simulink model "case8"  (R2024b)
settings: Solver=FixedStepAuto  StartTime=0  StopTime=1  FixedStep=1e-7  RelTol=1e-3
values from neighbouring files (symbols this model uses):
  SG_D_1_D = 0.01056    [IEEE9_case_parameters.m]    (also in case1_parameters.m; case2_parameters.m; case3_parameters.m; case4_parameters.m)
  SG_D_1_EnableSaturation = 0    [IEEE9_case_parameters.m]    (also in case1_parameters.m; case2_parameters.m; case3_parameters.m; case4_parameters.m)
  SG_D_1_f0 = 60    [IEEE9_case_parameters.m]    (also in case1_parameters.m; case2_parameters.m; case3_parameters.m; case4_parameters.m)
  SG_D_1_H = 7.5    [IEEE9_case_parameters.m]    (also in case1_parameters.m; case2_parameters.m; case3_parameters.m; case4_parameters.m)
  SG_D_1_K_A = 20    [IEEE9_case_parameters.m]    (also in case1_parameters.m; case2_parameters.m; case3_parameters.m; case4_parameters.m)
  SG_D_1_K_E = 1.000000e+1    (= 10)    [IEEE9_case_parameters.m]    (also in case1_parameters.m; case2_parameters.m; case3_parameters.m; case4_parameters.m)
  SG_D_1_K_F = 2.363    [IEEE9_case_parameters.m]    (also in case1_parameters.m; case2_parameters.m; case3_parameters.m; case4_parameters.m)
  SG_D_1_K_s = 0.5    [IEEE9_case_parameters.m]    (also in case1_parameters.m = 5; case2_parameters.m = 5; case3_parameters.m = 5; case4_parameters.m = 5)
  SG_D_1_R_a = 0.001088    [IEEE9_case_parameters.m]    (also in case1_parameters.m; case2_parameters.m; case3_parameters.m; case4_parameters.m)
  SG_D_1_S_A = 1    [IEEE9_case_parameters.m]    (also in case1_parameters.m; case2_parameters.m; case3_parameters.m; case4_parameters.m)
  SG_D_1_S_B = 0.103    [IEEE9_case_parameters.m]    (also in case1_parameters.m; case2_parameters.m; case3_parameters.m; case4_parameters.m)
  SG_D_1_S_N = 10.659857    [IEEE9_case_parameters.m]    (also in case1_parameters.m; case2_parameters.m; case3_parameters.m; case4_parameters.m)
  SG_D_1_SpeedPara = 200    [IEEE9_case_parameters.m]    (also in case1_parameters.m; case2_parameters.m; case3_parameters.m; case4_parameters.m)
  SG_D_1_T_0 = 0.720173    [IEEE9_case_parameters.m]    (also in case1_parameters.m = 0.755522; case2_parameters.m = 0.808931; case3_parameters.m = 0.869402; case4_parameters.m = 0.729316)
  SG_D_1_T_1 = 0.3    [IEEE9_case_parameters.m]    (also in case1_parameters.m; case2_parameters.m; case3_parameters.m; case4_parameters.m)
  SG_D_1_T_2 = 0.05    [IEEE9_case_parameters.m]    (also in case1_parameters.m; case2_parameters.m; case3_parameters.m; case4_parameters.m)
  SG_D_1_T_3 = 0.02    [IEEE9_case_parameters.m]    (also in case1_parameters.m; case2_parameters.m; case3_parameters.m; case4_parameters.m)
  SG_D_1_T_4 = 0.005    [IEEE9_case_parameters.m]    (also in case1_parameters.m; case2_parameters.m; case3_parameters.m; case4_parameters.m)
  SG_D_1_T_A = 0.02    [IEEE9_case_parameters.m]    (also in case1_parameters.m; case2_parameters.m; case3_parameters.m; case4_parameters.m)
  SG_D_1_T_dd = 8.000000e+0    (= 8)    [IEEE9_case_parameters.m]    (also in case1_parameters.m; case2_parameters.m; case3_parameters.m; case4_parameters.m)
  SG_D_1_T_ddd = 0.04    [IEEE9_case_parameters.m]    (also in case1_parameters.m; case2_parameters.m; case3_parameters.m; case4_parameters.m)
  SG_D_1_T_E = 0.314    [IEEE9_case_parameters.m]    (also in case1_parameters.m; case2_parameters.m; case3_parameters.m; case4_parameters.m)
  SG_D_1_T_F = 0.35    [IEEE9_case_parameters.m]    (also in case1_parameters.m; case2_parameters.m; case3_parameters.m; case4_parameters.m)
  SG_D_1_T_qd = 0.8    [IEEE9_case_parameters.m]    (also in case1_parameters.m; case2_parameters.m; case3_parameters.m; case4_parameters.m)
  SG_D_1_T_qdd = 0.02    [IEEE9_case_parameters.m]    (also in case1_parameters.m; case2_parameters.m; case3_parameters.m; case4_parameters.m)
  SG_D_1_T_speed = 0.1    [IEEE9_case_parameters.m]    (also in case1_parameters.m = 200; case2_parameters.m = 200; case3_parameters.m = 200; case4_parameters.m = 200)
  SG_D_1_T_w = 0.5    [IEEE9_case_parameters.m]    (also in case1_parameters.m; case2_parameters.m; case3_parameters.m; case4_parameters.m)
  SG_D_1_V_ref = 1.990276    [IEEE9_case_parameters.m]    (also in case1_parameters.m = 2.042296; case2_parameters.m = 2.051388; case3_parameters.m = 2.089584; case4_parameters.m = 2.01845)
  SG_D_1_w_ref = 376.991118    [IEEE9_case_parameters.m]    (also in case1_parameters.m; case2_parameters.m; case3_parameters.m; case4_parameters.m)
  SG_D_1_wb = 6.000000e+1    (= 60)    [IEEE9_case_parameters.m]    (also in case1_parameters.m; case2_parameters.m; case3_parameters.m; case4_parameters.m)
  SG_D_1_x_d = 1.9    [IEEE9_case_parameters.m]    (also in case1_parameters.m; case2_parameters.m; case3_parameters.m; case4_parameters.m)
  SG_D_1_x_dd = 0.302    [IEEE9_case_parameters.m]    (also in case1_parameters.m; case2_parameters.m; case3_parameters.m; case4_parameters.m)
  SG_D_1_x_ddd = 0.204    [IEEE9_case_parameters.m]    (also in case1_parameters.m; case2_parameters.m; case3_parameters.m; case4_parameters.m)
  SG_D_1_x_l = 0.05    [IEEE9_case_parameters.m]    (also in case1_parameters.m; case2_parameters.m; case3_parameters.m; case4_parameters.m)
  SG_D_1_x_q = 1.3    [IEEE9_case_parameters.m]    (also in case1_parameters.m; case2_parameters.m; case3_parameters.m; case4_parameters.m)
  SG_D_1_x_qd = 0.5    [IEEE9_case_parameters.m]    (also in case1_parameters.m; case2_parameters.m; case3_parameters.m; case4_parameters.m)
  SG_D_1_x_qdd = 0.3    [IEEE9_case_parameters.m]    (also in case1_parameters.m; case2_parameters.m; case3_parameters.m; case4_parameters.m)
  SG_D_2_D = 0.02    [IEEE9_case_parameters.m]    (also in case1_parameters.m; case2_parameters.m; case3_parameters.m; case4_parameters.m)
  SG_D_2_EnableSaturation = 0    [IEEE9_case_parameters.m]    (also in case1_parameters.m; case2_parameters.m; case3_parameters.m; case4_parameters.m)
  SG_D_2_f0 = 60    [IEEE9_case_parameters.m]    (also in case1_parameters.m; case2_parameters.m; case3_parameters.m; case4_parameters.m)
  SG_D_2_H = 8.000000e+0    (= 8)    [IEEE9_case_parameters.m]    (also in case1_parameters.m; case2_parameters.m; case3_parameters.m; case4_parameters.m)
  SG_D_2_K_A = 20    [IEEE9_case_parameters.m]    (also in case1_parameters.m; case2_parameters.m; case3_parameters.m; case4_parameters.m)
  SG_D_2_K_E = 1.000000e+1    (= 10)    [IEEE9_case_parameters.m]    (also in case1_parameters.m; case2_parameters.m; case3_parameters.m; case4_parameters.m)
  SG_D_2_K_F = 2.363    [IEEE9_case_parameters.m]    (also in case1_parameters.m; case2_parameters.m; case3_parameters.m; case4_parameters.m)
  SG_D_2_K_s = 0.5    [IEEE9_case_parameters.m]    (also in case1_parameters.m = 4; case2_parameters.m = 4; case3_parameters.m = 4; case4_parameters.m = 4)
  SG_D_2_R_a = 0.001088    [IEEE9_case_parameters.m]    (also in case1_parameters.m; case2_parameters.m; case3_parameters.m; case4_parameters.m)
  SG_D_2_S_A = 1    [IEEE9_case_parameters.m]    (also in case1_parameters.m; case2_parameters.m; case3_parameters.m; case4_parameters.m)
  SG_D_2_S_B = 0.103    [IEEE9_case_parameters.m]    (also in case1_parameters.m; case2_parameters.m; case3_parameters.m; case4_parameters.m)
  SG_D_2_S_N = 10.659857    [IEEE9_case_parameters.m]    (also in case1_parameters.m; case2_parameters.m; case3_parameters.m; case4_parameters.m)
  SG_D_2_SpeedPara = 200    [IEEE9_case_parameters.m]    (also in case1_parameters.m; case2_parameters.m; case3_parameters.m; case4_parameters.m)
  SG_D_2_T_0 = 1.632913    [IEEE9_case_parameters.m]    (also in case1_parameters.m = 1.632925; case2_parameters.m = 1.632915; case3_parameters.m = 1.632914; case4_parameters.m = 1.632927)
  SG_D_2_T_1 = 0.2    [IEEE9_case_parameters.m]    (also in case1_parameters.m; case2_parameters.m; case3_parameters.m; case4_parameters.m)
  SG_D_2_T_2 = 0.05    [IEEE9_case_parameters.m]    (also in case1_parameters.m; case2_parameters.m; case3_parameters.m; case4_parameters.m)
  SG_D_2_T_3 = 0.02    [IEEE9_case_parameters.m]    (also in case1_parameters.m; case2_parameters.m; case3_parameters.m; case4_parameters.m)
  SG_D_2_T_4 = 0.005    [IEEE9_case_parameters.m]    (also in case1_parameters.m; case2_parameters.m; case3_parameters.m; case4_parameters.m)
  SG_D_2_T_A = 0.02    [IEEE9_case_parameters.m]    (also in case1_parameters.m; case2_parameters.m; case3_parameters.m; case4_parameters.m)
  SG_D_2_T_dd = 7.9    [IEEE9_case_parameters.m]    (also in case1_parameters.m; case2_parameters.m; case3_parameters.m; case4_parameters.m)
  SG_D_2_T_ddd = 0.04    [IEEE9_case_parameters.m]    (also in case1_parameters.m; case2_parameters.m; case3_parameters.m; case4_parameters.m)
  SG_D_2_T_E = 0.314    [IEEE9_case_parameters.m]    (also in case1_parameters.m; case2_parameters.m; case3_parameters.m; case4_parameters.m)
  SG_D_2_T_F = 0.35    [IEEE9_case_parameters.m]    (also in case1_parameters.m; case2_parameters.m; case3_parameters.m; case4_parameters.m)
  SG_D_2_T_qd = 0.8    [IEEE9_case_parameters.m]    (also in case1_parameters.m; case2_parameters.m; case3_parameters.m; case4_parameters.m)
  SG_D_2_T_qdd = 0.015    [IEEE9_case_parameters.m]    (also in case1_parameters.m; case2_parameters.m; case3_parameters.m; case4_parameters.m)
  SG_D_2_T_speed = 0.1    [IEEE9_case_parameters.m]    (also in case1_parameters.m = 150; case2_parameters.m = 150; case3_parameters.m = 150; case4_parameters.m = 150)
  SG_D_2_T_w = 0.35    [IEEE9_case_parameters.m]    (also in case1_parameters.m; case2_parameters.m; case3_parameters.m; case4_parameters.m)
  SG_D_2_V_ref = 2.58547    [IEEE9_case_parameters.m]    (also in case1_parameters.m = 2.597896; case2_parameters.m = 2.587136; case3_parameters.m = 2.586042; case4_parameters.m = 2.599679)
  SG_D_2_w_ref = 376.991118    [IEEE9_case_parameters.m]    (also in case1_parameters.m; case2_parameters.m; case3_parameters.m; case4_parameters.m)
  SG_D_2_wb = 6.000000e+1    (= 60)    [IEEE9_case_parameters.m]    (also in case1_parameters.m; case2_parameters.m; case3_parameters.m; case4_parameters.m)
  SG_D_2_x_d = 1.8    [IEEE9_case_parameters.m]    (also in case1_parameters.m; case2_parameters.m; case3_parameters.m; case4_parameters.m)
  SG_D_2_x_dd = 0.302    [IEEE9_case_parameters.m]    (also in case1_parameters.m; case2_parameters.m; case3_parameters.m; case4_parameters.m)
  SG_D_2_x_ddd = 0.204    [IEEE9_case_parameters.m]    (also in case1_parameters.m; case2_parameters.m; case3_parameters.m; case4_parameters.m)
  SG_D_2_x_l = 0.05    [IEEE9_case_parameters.m]    (also in case1_parameters.m; case2_parameters.m; case3_parameters.m; case4_parameters.m)
  SG_D_2_x_q = 1.25    [IEEE9_case_parameters.m]    (also in case1_parameters.m; case2_parameters.m; case3_parameters.m; case4_parameters.m)
  SG_D_2_x_qd = 0.5    [IEEE9_case_parameters.m]    (also in case1_parameters.m; case2_parameters.m; case3_parameters.m; case4_parameters.m)
  SG_D_2_x_qdd = 0.3    [IEEE9_case_parameters.m]    (also in case1_parameters.m; case2_parameters.m; case3_parameters.m; case4_parameters.m)
  SG_D_3_D = 0.02    [IEEE9_case_parameters.m]    (also in case1_parameters.m; case2_parameters.m; case3_parameters.m; case4_parameters.m)
  SG_D_3_EnableSaturation = 0    [IEEE9_case_parameters.m]    (also in case1_parameters.m; case2_parameters.m; case3_parameters.m; case4_parameters.m)
  SG_D_3_f0 = 60    [IEEE9_case_parameters.m]    (also in case1_parameters.m; case2_parameters.m; case3_parameters.m; case4_parameters.m)
  SG_D_3_H = 7.7    [IEEE9_case_parameters.m]    (also in case1_parameters.m; case2_parameters.m; case3_parameters.m; case4_parameters.m)
  SG_D_3_K_A = 20    [IEEE9_case_parameters.m]    (also in case1_parameters.m; case2_parameters.m; case3_parameters.m; case4_parameters.m)
  SG_D_3_K_E = 1.000000e+1    (= 10)    [IEEE9_case_parameters.m]    (also in case1_parameters.m; case2_parameters.m; case3_parameters.m; case4_parameters.m)
  SG_D_3_K_F = 2.363    [IEEE9_case_parameters.m]    (also in case1_parameters.m; case2_parameters.m; case3_parameters.m; case4_parameters.m)
  SG_D_3_K_s = 0.2    [IEEE9_case_parameters.m]    (also in case1_parameters.m = 2; case2_parameters.m = 2; case3_parameters.m = 2; case4_parameters.m = 2)
  SG_D_3_R_a = 0.001088    [IEEE9_case_parameters.m]    (also in case1_parameters.m; case2_parameters.m; case3_parameters.m; case4_parameters.m)
  SG_D_3_S_A = 1    [IEEE9_case_parameters.m]    (also in case1_parameters.m; case2_parameters.m; case3_parameters.m; case4_parameters.m)
  SG_D_3_S_B = 0.103    [IEEE9_case_parameters.m]    (also in case1_parameters.m; case2_parameters.m; case3_parameters.m; case4_parameters.m)
  SG_D_3_S_N = 10.659857    [IEEE9_case_parameters.m]    (also in case1_parameters.m; case2_parameters.m; case3_parameters.m; case4_parameters.m)
  SG_D_3_SpeedPara = 200    [IEEE9_case_parameters.m]    (also in case1_parameters.m; case2_parameters.m; case3_parameters.m; case4_parameters.m)
  SG_D_3_T_0 = 0.850788    [IEEE9_case_parameters.m]    (also in case1_parameters.m = 0.850786; case2_parameters.m = 0.850787; case3_parameters.m; case4_parameters.m = 0.850786)
  SG_D_3_T_1 = 0.2    [IEEE9_case_parameters.m]    (also in case1_parameters.m; case2_parameters.m; case3_parameters.m; case4_parameters.m)
  SG_D_3_T_2 = 0.05    [IEEE9_case_parameters.m]    (also in case1_parameters.m; case2_parameters.m; case3_parameters.m; case4_parameters.m)
  SG_D_3_T_3 = 0.02    [IEEE9_case_parameters.m]    (also in case1_parameters.m; case2_parameters.m; case3_parameters.m; case4_parameters.m)
  SG_D_3_T_4 = 0.005    [IEEE9_case_parameters.m]    (also in case1_parameters.m; case2_parameters.m; case3_parameters.m; case4_parameters.m)
  SG_D_3_T_A = 0.02    [IEEE9_case_parameters.m]    (also in case1_parameters.m; case2_parameters.m; case3_parameters.m; case4_parameters.m)
  SG_D_3_T_dd = 8.1    [IEEE9_case_parameters.m]    (also in case1_parameters.m; case2_parameters.m; case3_parameters.m; case4_parameters.m)
  SG_D_3_T_ddd = 0.04    [IEEE9_case_parameters.m]    (also in case1_parameters.m; case2_parameters.m; case3_parameters.m; case4_parameters.m)
  SG_D_3_T_E = 0.314    [IEEE9_case_parameters.m]    (also in case1_parameters.m; case2_parameters.m; case3_parameters.m; case4_parameters.m)
  SG_D_3_T_F = 0.35    [IEEE9_case_parameters.m]    (also in case1_parameters.m; case2_parameters.m; case3_parameters.m; case4_parameters.m)
  SG_D_3_T_qd = 0.8    [IEEE9_case_parameters.m]    (also in case1_parameters.m; case2_parameters.m; case3_parameters.m; case4_parameters.m)
  SG_D_3_T_qdd = 0.015    [IEEE9_case_parameters.m]    (also in case1_parameters.m; case2_parameters.m; case3_parameters.m; case4_parameters.m)
  SG_D_3_T_speed = 0.1    [IEEE9_case_parameters.m]    (also in case1_parameters.m = 180; case2_parameters.m = 180; case3_parameters.m = 180; case4_parameters.m = 180)
  SG_D_3_T_w = 0.4    [IEEE9_case_parameters.m]    (also in case1_parameters.m; case2_parameters.m; case3_parameters.m; case4_parameters.m)
  SG_D_3_V_ref = 1.892727    [IEEE9_case_parameters.m]    (also in case1_parameters.m = 1.906439; case2_parameters.m = 1.895535; case3_parameters.m = 1.892105; case4_parameters.m = 1.906598)
  SG_D_3_w_ref = 376.991118    [IEEE9_case_parameters.m]    (also in case1_parameters.m; case2_parameters.m; case3_parameters.m; case4_parameters.m)
  SG_D_3_wb = 6.000000e+1    (= 60)    [IEEE9_case_parameters.m]    (also in case1_parameters.m; case2_parameters.m; case3_parameters.m; case4_parameters.m)
  SG_D_3_x_d = 1.85    [IEEE9_case_parameters.m]    (also in case1_parameters.m; case2_parameters.m; case3_parameters.m; case4_parameters.m)
  SG_D_3_x_dd = 0.302    [IEEE9_case_parameters.m]    (also in case1_parameters.m; case2_parameters.m; case3_parameters.m; case4_parameters.m)
  SG_D_3_x_ddd = 0.204    [IEEE9_case_parameters.m]    (also in case1_parameters.m; case2_parameters.m; case3_parameters.m; case4_parameters.m)
  SG_D_3_x_l = 0.05    [IEEE9_case_parameters.m]    (also in case1_parameters.m; case2_parameters.m; case3_parameters.m; case4_parameters.m)
  SG_D_3_x_q = 1.2    [IEEE9_case_parameters.m]    (also in case1_parameters.m; case2_parameters.m; case3_parameters.m; case4_parameters.m)
  SG_D_3_x_qd = 0.5    [IEEE9_case_parameters.m]    (also in case1_parameters.m; case2_parameters.m; case3_parameters.m; case4_parameters.m)
  SG_D_3_x_qdd = 0.3    [IEEE9_case_parameters.m]    (also in case1_parameters.m; case2_parameters.m; case3_parameters.m; case4_parameters.m)
(part 5 of 12)

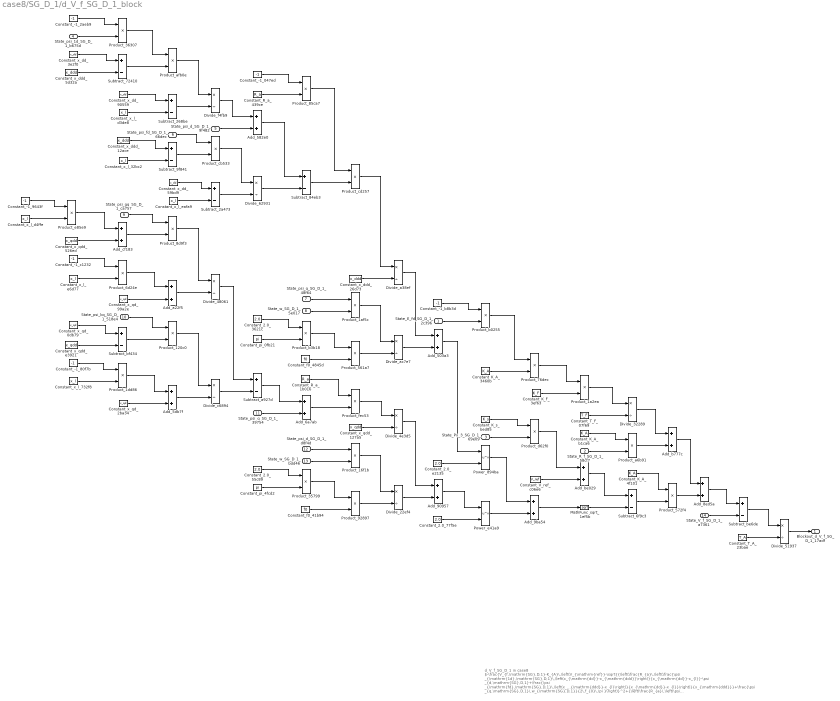
== system case8/SG_D_1/d_V_f_SG_D_1_block ==
  note: d_V_f_SG_D_1 in case8
      | $-\frac{V_{f,\mathrm{SG},D,1}-K_{A}\,\left(V_{\mathrm{ref}}-\sqrt{{\left(\frac{R_{a}\,\left(\frac{\psi _{\mathrm{1d},\mathrm{SG},D,1}\,\left(x_{\mathrm{dd}}-x_{\mathrm{ddd}}\right)}{x_{\mathrm{dd}}-x_{l}}-\psi _{d,\mathrm{SG},D,1}+\frac{\psi _{\mathrm{fd},\mathrm{SG},D,1}\,\left(x_{\mathrm{ddd}}-x_{l}\right)}{x_{\mathrm{dd}}-x_{l}}\right)}{x_{\mathrm{ddd}}}+\frac{\psi _{q,\mathrm{SG},D,1}\,w_{\mathrm{SG},D,1}}{2\,f_{0}\,\pi }\right)}^2+{\left(\frac{R_{a}\,\left(\psi _{q,\mathrm{SG},D,1}+\frac{\psi _{\mathrm{gq},\mathrm{SG},D,1}\,\left(x_{l}-x_{\mathrm{qdd}}\right)}{x_{l}-x_{\mathrm{qd}}}+\frac{\psi _{\mathrm{kq},\mathrm{SG},D,1}\,\left(x_{\mathrm{qd}}-x_{\mathrm{qdd}}\right)}{x_{l}-x_{\mathrm{qd}}}\right)}{x_{\mathrm{qdd}}}+\frac{\psi _{d,\mathrm{SG},D,1}\,w_{\mathrm{SG},D,1}}{2\,f_{0}\,\pi }\right)}^2}+K_{s}\,\mathrm{Px}_{3,\mathrm{SG},D,1}\right)-K_{A}\,R_{f,\mathrm{SG},D,1}+\frac{E_{\mathrm{fd},\mathrm{SG},D,1}\,K_{A}\,K_{F}}{T_{F}}}{T_{A}}$
      | Automatically generated on 2025-10-31 19:29:38 .
  State_E_fd_SG_D_1_2c396 : Inport
  State_R_f_SG_D_1_58cf7 : Inport  Port=2
  State_Px_3_SG_D_1_69e09 : Inport  Port=3
  State_psi_1d_SG_D_1_b675d : Inport  Port=4
  State_psi_d_SG_D_1_9f482 : Inport  Port=5
  State_psi_fd_SG_D_1_66dec : Inport  Port=6
  State_psi_q_SG_D_1_48f64 : Inport  Port=7
  State_w_SG_D_1_5e017 : Inport  Port=8
  State_psi_gq_SG_D_1_ca757 : Inport  Port=9
  State_psi_kq_SG_D_1_518e4 : Inport  Port=10
  State_psi_q_SG_D_1_39754 : Inport  Port=11
  State_psi_d_SG_D_1_d8f4d : Inport  Port=12
  State_w_SG_D_1_bdd46 : Inport  Port=13
  State_V_f_SG_D_1_a7361 : Inport  Port=14
  Add_503a3 : Sum
  Add_582e0 : Sum
  Add_5db7f : Sum
  Add_6a7ab : Sum
  Add_8ed5a : Sum
  Add_90957 : Sum
  Add_9ba54 : Sum
  Add_a22f5 : Sum
  Add_b777c : Sum
  Add_be029 : Sum
  Add_cf183 : Sum
  Constant_-1_047ed : Constant  Value=-1
  Constant_-1_2aeb9 : Constant  Value=-1
  Constant_-1_80f7b : Constant  Value=-1
  Constant_-1_9643f : Constant  Value=-1
  Constant_-1_b8b3d : Constant  Value=-1
  Constant_-1_c1232 : Constant  Value=-1
  Constant_2.0_3621c : Constant  Value=2.0
  Constant_2.0_55c89 : Constant  Value=2.0
  Constant_2.0_77f5e : Constant  Value=2.0
  Constant_2.0_e2135 : Constant  Value=2.0
  Constant_K_A_3460b : Constant  Value=K_A
  Constant_K_A_4f101 : Constant  Value=K_A
  Constant_K_A_b1ca6 : Constant  Value=K_A
  Constant_K_F_3ef63 : Constant  Value=K_F
  Constant_K_s_bed85 : Constant  Value=K_s
  Constant_R_a_1b016 : Constant  Value=R_a
  Constant_R_a_439ce : Constant  Value=R_a
  Constant_T_A_23bae : Constant  Value=T_A
  Constant_T_F_07f69 : Constant  Value=T_F
  Constant_V_ref_c06e6 : Constant  Value=V_ref
  Constant_f0_41b94 : Constant  Value=f0
  Constant_f0_4845d : Constant  Value=f0
  Constant_pi_0fb21 : Constant  Value=pi
  Constant_pi_4fcd2 : Constant  Value=pi
  Constant_x_dd_3e2f0 : Constant  Value=x_dd
  Constant_x_dd_59bd9 : Constant  Value=x_dd
  Constant_x_dd_90559 : Constant  Value=x_dd
  Constant_x_ddd_12ace : Constant  Value=x_ddd
  Constant_x_ddd_26d73 : Constant  Value=x_ddd
  Constant_x_ddd_5d32a : Constant  Value=x_ddd
  Constant_x_l_32bc2 : Constant  Value=x_l
  Constant_x_l_732f8 : Constant  Value=x_l
  Constant_x_l_d3de8 : Constant  Value=x_l
  Constant_x_l_d4ffe : Constant  Value=x_l
  Constant_x_l_e6d77 : Constant  Value=x_l
  Constant_x_l_eafa9 : Constant  Value=x_l
  Constant_x_qd_0db79 : Constant  Value=x_qd
  Constant_x_qd_2ba34 : Constant  Value=x_qd
  Constant_x_qd_99a2e : Constant  Value=x_qd
  Constant_x_qdd_127a5 : Constant  Value=x_qdd
  Constant_x_qdd_526ed : Constant  Value=x_qdd
  Constant_x_qdd_e3921 : Constant  Value=x_qdd
  Divide_22ef4 : Product  Inputs=*/
  Divide_{32289,48061,51937,62931} (4 alike) : Product  Inputs=*/
  Divide_4e3d5 : Product  Inputs=*/
  Divide_a38ef : Product  Inputs=*/
  Divide_ac7e7 : Product  Inputs=*/
  Divide_c6894 : Product  Inputs=*/
  Divide_f4fb9 : Product  Inputs=*/
  MathFunc_sqrt_1ef5b : Sqrt
  Power_894ba : Math  Operator=pow
  Power_e41a9 : Math  Operator=pow
  Product_120c0 : Product
  Product_16f1b : Product
  Product_1a2ea : Product
  Product_1af5c : Product
  Product_1dd86 : Product
  Product_35799 : Product
  Product_36307 : Product
  Product_561a7 : Product
  Product_572f4 : Product
  Product_6d24e : Product
  Product_76dec : Product
  Product_85ca7 : Product
  Product_8d9f3 : Product
  Product_92897 : Product
  Product_a6b91 : Product
  Product_afb0e : Product
  Product_b0255 : Product
  Product_b3b18 : Product
  Product_cb533 : Product
  Product_cd257 : Product
  Product_d62f0 : Product
  Product_e85e9 : Product
  Product_fec53 : Product
  Subtract_268be : Sum  Inputs=+-
  Subtract_2a473 : Sum  Inputs=+-
  Subtract_6f9c3 : Sum  Inputs=+-
  Subtract_72410 : Sum  Inputs=+-
  Subtract_84eb3 : Sum  Inputs=+-
  Subtract_9f841 : Sum  Inputs=+-
  Subtract_a927d : Sum  Inputs=+-
  Subtract_be6de : Sum  Inputs=+-
  Subtract_bf434 : Sum  Inputs=+-
  Blockout_d_V_f_SG_D_1_17adf : Outport
  wires:
  Constant_-1_80f7b/1 -> Product_1dd86/1
  Constant_-1_9643f/1 -> Product_e85e9/1
  State_psi_d_SG_D_1_d8f4d/1 -> Product_16f1b/1
  Constant_x_qd_2ba34/1 -> Add_5db7f/2
  Constant_x_qdd_526ed/1 -> Add_cf183/2
  State_w_SG_D_1_bdd46/1 -> Product_16f1b/2
  Constant_x_l_d4ffe/1 -> Product_e85e9/2
  Subtract_84eb3/1 -> Product_cd257/2
  Constant_x_l_732f8/1 -> Product_1dd86/2
  Constant_x_dd_3e2f0/1 -> Subtract_72410/1
  Constant_R_a_439ce/1 -> Product_85ca7/2
  Constant_-1_2aeb9/1 -> Product_36307/1
  Divide_62931/1 -> Subtract_84eb3/2
  Constant_x_ddd_5d32a/1 -> Subtract_72410/2
  Add_5db7f/1 -> Divide_c6894/2
  State_psi_1d_SG_D_1_b675d/1 -> Product_36307/2
  Add_a22f5/1 -> Divide_48061/2
  Subtract_bf434/1 -> Product_120c0/2
  Product_1a2ea/1 -> Divide_32289/1
  Product_b3b18/1 -> Product_561a7/1
  Product_e85e9/1 -> Add_cf183/1
  Constant_-1_c1232/1 -> Product_6d24e/1
  Constant_x_l_e6d77/1 -> Product_6d24e/2
  Add_582e0/1 -> Subtract_84eb3/1
  Constant_2.0_55c89/1 -> Product_35799/1
  Constant_x_qd_0db79/1 -> Subtract_bf434/1
  Product_36307/1 -> Product_afb0e/1
  Constant_pi_4fcd2/1 -> Product_35799/2
  Constant_x_qdd_e3921/1 -> Subtract_bf434/2
  Subtract_72410/1 -> Product_afb0e/2
  State_psi_q_SG_D_1_39754/1 -> Add_6a7ab/2
  Constant_x_dd_90559/1 -> Subtract_268be/1
  Constant_x_l_d3de8/1 -> Subtract_268be/2
  Constant_x_ddd_12ace/1 -> Subtract_9f841/1
  Constant_x_l_32bc2/1 -> Subtract_9f841/2
  State_psi_gq_SG_D_1_ca757/1 -> Product_8d9f3/1
  Add_cf183/1 -> Product_8d9f3/2
  Product_6d24e/1 -> Add_a22f5/1
  Constant_x_qd_99a2e/1 -> Add_a22f5/2
  Divide_f4fb9/1 -> Add_582e0/1
  Subtract_268be/1 -> Divide_f4fb9/2
  State_psi_kq_SG_D_1_518e4/1 -> Product_120c0/1
  Divide_51937/1 -> Blockout_d_V_f_SG_D_1_17adf/1
  Product_1dd86/1 -> Add_5db7f/1
  Product_afb0e/1 -> Divide_f4fb9/1
  State_psi_fd_SG_D_1_66dec/1 -> Product_cb533/1
  State_w_SG_D_1_5e017/1 -> Product_1af5c/2
  Subtract_9f841/1 -> Product_cb533/2
  Constant_x_dd_59bd9/1 -> Subtract_2a473/1
  Constant_x_l_eafa9/1 -> Subtract_2a473/2
  Product_8d9f3/1 -> Divide_48061/1
  Product_85ca7/1 -> Product_cd257/1
  Product_120c0/1 -> Divide_c6894/1
  State_psi_d_SG_D_1_9f482/1 -> Add_582e0/2
  Product_cb533/1 -> Divide_62931/1
  Subtract_2a473/1 -> Divide_62931/2
  Divide_48061/1 -> Subtract_a927d/1
  Divide_c6894/1 -> Subtract_a927d/2
  Constant_-1_047ed/1 -> Product_85ca7/1
  Constant_2.0_3621c/1 -> Product_b3b18/1
  Constant_pi_0fb21/1 -> Product_b3b18/2
  Subtract_a927d/1 -> Add_6a7ab/1
  State_psi_q_SG_D_1_48f64/1 -> Product_1af5c/1
  Constant_f0_4845d/1 -> Product_561a7/2
  Constant_R_a_1b016/1 -> Product_fec53/1
  Add_6a7ab/1 -> Product_fec53/2
  Product_35799/1 -> Product_92897/1
  Power_894ba/1 -> Add_9ba54/1
  Constant_f0_41b94/1 -> Product_92897/2
  Product_cd257/1 -> Divide_a38ef/1
  Constant_x_ddd_26d73/1 -> Divide_a38ef/2
  Product_1af5c/1 -> Divide_ac7e7/1
  Product_561a7/1 -> Divide_ac7e7/2
  Product_fec53/1 -> Divide_4e3d5/1
  Constant_x_qdd_127a5/1 -> Divide_4e3d5/2
  Product_16f1b/1 -> Divide_22ef4/1
  Product_92897/1 -> Divide_22ef4/2
  Divide_a38ef/1 -> Add_503a3/1
  Divide_ac7e7/1 -> Add_503a3/2
  Divide_4e3d5/1 -> Add_90957/1
  Divide_22ef4/1 -> Add_90957/2
  Constant_-1_b8b3d/1 -> Product_b0255/1
  State_E_fd_SG_D_1_2c396/1 -> Product_b0255/2
  Add_503a3/1 -> Power_894ba/1
  Constant_2.0_e2135/1 -> Power_894ba/2
  Add_90957/1 -> Power_e41a9/1
  Constant_2.0_77f5e/1 -> Power_e41a9/2
  Product_b0255/1 -> Product_76dec/1
  Constant_K_A_3460b/1 -> Product_76dec/2
  Constant_K_s_bed85/1 -> Product_d62f0/1
  State_Px_3_SG_D_1_69e09/1 -> Product_d62f0/2
  Power_e41a9/1 -> Add_9ba54/2
  Divide_32289/1 -> Add_b777c/1
  Product_76dec/1 -> Product_1a2ea/1
  Constant_K_F_3ef63/1 -> Product_1a2ea/2
  Product_d62f0/1 -> Add_be029/1
  Constant_V_ref_c06e6/1 -> Add_be029/2
  Add_9ba54/1 -> MathFunc_sqrt_1ef5b/1
  Constant_T_F_07f69/1 -> Divide_32289/2
  Constant_K_A_b1ca6/1 -> Product_a6b91/1
  State_R_f_SG_D_1_58cf7/1 -> Product_a6b91/2
  Add_be029/1 -> Subtract_6f9c3/1
  MathFunc_sqrt_1ef5b/1 -> Subtract_6f9c3/2
  Constant_T_A_23bae/1 -> Divide_51937/2
  Product_a6b91/1 -> Add_b777c/2
  Constant_K_A_4f101/1 -> Product_572f4/1
  Subtract_6f9c3/1 -> Product_572f4/2
  Add_b777c/1 -> Add_8ed5a/1
  Product_572f4/1 -> Add_8ed5a/2
  Add_8ed5a/1 -> Subtract_be6de/1
  State_V_f_SG_D_1_a7361/1 -> Subtract_be6de/2
  Subtract_be6de/1 -> Divide_51937/1

== system case8/SG_D_1/d_psi_1d_SG_D_1_block ==
  note: d_psi_1d_SG_D_1 in case8
      | $-\frac{\psi _{\mathrm{1d},\mathrm{SG},D,1}-\psi _{\mathrm{fd},\mathrm{SG},D,1}+\frac{\left(x_{\mathrm{dd}}-x_{l}\right)\,\left(\frac{\psi _{\mathrm{1d},\mathrm{SG},D,1}\,\left(x_{\mathrm{dd}}-x_{\mathrm{ddd}}\right)}{x_{\mathrm{dd}}-x_{l}}-\psi _{d,\mathrm{SG},D,1}+\frac{\psi _{\mathrm{fd},\mathrm{SG},D,1}\,\left(x_{\mathrm{ddd}}-x_{l}\right)}{x_{\mathrm{dd}}-x_{l}}\right)}{x_{\mathrm{ddd}}}}{T_{\mathrm{ddd}}}$
      | Automatically generated on 2025-10-31 19:29:32 .
  State_psi_1d_SG_D_1_47359 : Inport
  State_psi_fd_SG_D_1_06edd : Inport  Port=2
  State_psi_1d_SG_D_1_6c7ce : Inport  Port=3
  State_psi_d_SG_D_1_372e8 : Inport  Port=4
  State_psi_fd_SG_D_1_43462 : Inport  Port=5
  Add_36161 : Sum
  Add_906ad : Sum
  Add_a494f : Sum
  Constant_-1_8beaa : Constant  Value=-1
  Constant_-1_a69bc : Constant  Value=-1
  Constant_T_ddd_2d7a7 : Constant  Value=T_ddd
  Constant_x_dd_747d7 : Constant  Value=x_dd
  Constant_x_dd_8f849 : Constant  Value=x_dd
  Constant_x_dd_b9147 : Constant  Value=x_dd
  Constant_x_dd_cba57 : Constant  Value=x_dd
  Constant_x_ddd_7197e : Constant  Value=x_ddd
  Constant_x_ddd_b6710 : Constant  Value=x_ddd
  Constant_x_ddd_c6c40 : Constant  Value=x_ddd
  Constant_x_l_05e27 : Constant  Value=x_l
  Constant_x_l_2042a : Constant  Value=x_l
  Constant_x_l_c0dd9 : Constant  Value=x_l
  Constant_x_l_cc2b8 : Constant  Value=x_l
  Divide_6006a : Product  Inputs=*/
  Divide_869c3 : Product  Inputs=*/
  Divide_ec7dd : Product  Inputs=*/
  Divide_fb428 : Product  Inputs=*/
  Product_216b7 : Product
  Product_34d88 : Product
  Product_969cd : Product
  Product_9cdaa : Product
  Product_e614f : Product
  Subtract_311db : Sum  Inputs=+-
  Subtract_6b82a : Sum  Inputs=+-
  Subtract_70435 : Sum  Inputs=+-
  Subtract_777bf : Sum  Inputs=+-
  Subtract_9e938 : Sum  Inputs=+-
  Subtract_a6006 : Sum  Inputs=+-
  Blockout_d_psi_1d_SG_D_1_a3e0f : Outport
  wires:
  Product_e614f/1 -> Product_9cdaa/1
  Constant_-1_a69bc/1 -> Product_e614f/1
  Subtract_311db/1 -> Product_9cdaa/2
  State_psi_1d_SG_D_1_6c7ce/1 -> Product_e614f/2
  Subtract_a6006/1 -> Product_216b7/1
  State_psi_d_SG_D_1_372e8/1 -> Add_a494f/2
  Constant_x_dd_747d7/1 -> Subtract_777bf/1
  Constant_x_l_c0dd9/1 -> Subtract_a6006/2
  Constant_x_dd_cba57/1 -> Subtract_311db/1
  Subtract_70435/1 -> Product_34d88/2
  Constant_x_l_2042a/1 -> Subtract_777bf/2
  Divide_ec7dd/1 -> Subtract_9e938/2
  Constant_x_ddd_b6710/1 -> Subtract_311db/2
  Constant_x_ddd_7197e/1 -> Subtract_70435/1
  Constant_x_l_05e27/1 -> Subtract_70435/2
  Add_906ad/1 -> Add_36161/1
  Product_9cdaa/1 -> Divide_fb428/1
  Divide_6006a/1 -> Add_36161/2
  Subtract_777bf/1 -> Divide_fb428/2
  State_psi_fd_SG_D_1_43462/1 -> Product_34d88/1
  Constant_x_dd_b9147/1 -> Subtract_6b82a/1
  Constant_x_l_cc2b8/1 -> Subtract_6b82a/2
  Constant_x_ddd_c6c40/1 -> Divide_6006a/2
  Subtract_9e938/1 -> Product_216b7/2
  Divide_fb428/1 -> Add_a494f/1
  Product_34d88/1 -> Divide_ec7dd/1
  Subtract_6b82a/1 -> Divide_ec7dd/2
  Product_216b7/1 -> Divide_6006a/1
  Constant_x_dd_8f849/1 -> Subtract_a6006/1
  Add_a494f/1 -> Subtract_9e938/1
  Constant_-1_8beaa/1 -> Product_969cd/1
  State_psi_1d_SG_D_1_47359/1 -> Product_969cd/2
  Product_969cd/1 -> Add_906ad/1
  State_psi_fd_SG_D_1_06edd/1 -> Add_906ad/2
  Add_36161/1 -> Divide_869c3/1
  Constant_T_ddd_2d7a7/1 -> Divide_869c3/2
  Divide_869c3/1 -> Blockout_d_psi_1d_SG_D_1_a3e0f/1

== system case8/SG_D_1/d_psi_d_SG_D_1_block ==
  note: d_psi_d_SG_D_1 in case8
      | $2\,\pi \,f_{0}\,\left(v_{d,\mathrm{SG},D,1}\,\sin\left(\theta _{\mathrm{SG},D,1}\right)-v_{q,\mathrm{SG},D,1}\,\cos\left(\theta _{\mathrm{SG},D,1}\right)+\frac{R_{a}\,\left(\frac{\psi _{\mathrm{1d},\mathrm{SG},D,1}\,\left(x_{\mathrm{dd}}-x_{\mathrm{ddd}}\right)}{x_{\mathrm{dd}}-x_{l}}-\psi _{d,\mathrm{SG},D,1}+\frac{\psi _{\mathrm{fd},\mathrm{SG},D,1}\,\left(x_{\mathrm{ddd}}-x_{l}\right)}{x_{\mathrm{dd}}-x_{l}}\right)}{x_{\mathrm{ddd}}}+\frac{\psi _{q,\mathrm{SG},D,1}\,w_{\mathrm{SG},D,1}}{2\,f_{0}\,\pi }\right)$
      | Automatically generated on 2025-10-31 19:29:26 .
  State_psi_1d_SG_D_1_0a3f1 : Inport
  State_psi_d_SG_D_1_d3b6a : Inport  Port=2
  State_psi_fd_SG_D_1_4a659 : Inport  Port=3
  Input_v_d_SG_D_1_7e265 : Inport  Port=4
  State_theta_SG_D_1_684aa : Inport  Port=5
  Input_v_q_SG_D_1_b5510 : Inport  Port=6
  State_theta_SG_D_1_1ab10 : Inport  Port=7
  State_psi_q_SG_D_1_546c2 : Inport  Port=8
  State_w_SG_D_1_cd758 : Inport  Port=9
  Add_625df : Sum
  Add_6e619 : Sum
  Constant_-1_be99b : Constant  Value=-1
  Constant_-2.0_2801a : Constant  Value=-2.0
  Constant_2.0_7bc02 : Constant  Value=2.0
  Constant_R_a_a2592 : Constant  Value=R_a
  Constant_f0_18599 : Constant  Value=f0
  Constant_f0_5b7b8 : Constant  Value=f0
  Constant_pi_56cff : Constant  Value=pi
  Constant_pi_e16f2 : Constant  Value=pi
  Constant_x_dd_3614c : Constant  Value=x_dd
  Constant_x_dd_e20fa : Constant  Value=x_dd
  Constant_x_dd_fa04e : Constant  Value=x_dd
  Constant_x_ddd_058ab : Constant  Value=x_ddd
  Constant_x_ddd_209e2 : Constant  Value=x_ddd
  Constant_x_ddd_e0a23 : Constant  Value=x_ddd
  Constant_x_l_35342 : Constant  Value=x_l
  Constant_x_l_6bd17 : Constant  Value=x_l
  Constant_x_l_ebb71 : Constant  Value=x_l
  Divide_04fac : Product  Inputs=*/
  Divide_1490a : Product  Inputs=*/
  Divide_39bf3 : Product  Inputs=*/
  Divide_a7949 : Product  Inputs=*/
  MathFunc_cos_ec301 : Trigonometry  Operator=cos
  MathFunc_sin_a89c5 : Trigonometry
  Product_073ea : Product
  Product_0a1c5 : Product
  Product_136b1 : Product
  Product_16869 : Product
  Product_74c8c : Product
  Product_8bf94 : Product
  Product_a81f3 : Product
  Product_aa5e2 : Product
  Product_b0c62 : Product
  Product_b9ea6 : Product
  Product_dfdca : Product
  Product_e62b2 : Product
  Subtract_660a1 : Sum  Inputs=+-
  Subtract_6b787 : Sum  Inputs=+-
  Subtract_834dc : Sum  Inputs=+-
  Subtract_9f2d1 : Sum  Inputs=+-
  Subtract_aaa06 : Sum  Inputs=+-
  Subtract_bd479 : Sum  Inputs=+-
  Subtract_e8463 : Sum  Inputs=+-
  Blockout_d_psi_d_SG_D_1_08662 : Outport
  wires:
  Add_6e619/1 -> Subtract_aaa06/1
  Product_16869/1 -> Divide_a7949/1
  Subtract_660a1/1 -> Product_16869/2
  Divide_a7949/1 -> Add_6e619/1
  Product_136b1/1 -> Product_16869/1
  Constant_x_ddd_e0a23/1 -> Subtract_660a1/2
  Constant_x_dd_e20fa/1 -> Subtract_660a1/1
  State_psi_1d_SG_D_1_0a3f1/1 -> Product_136b1/2
  Constant_-1_be99b/1 -> Product_136b1/1
  Product_aa5e2/1 -> Divide_39bf3/1
  Constant_x_l_ebb71/1 -> Subtract_bd479/2
  State_psi_d_SG_D_1_d3b6a/1 -> Add_6e619/2
  Constant_x_dd_fa04e/1 -> Subtract_bd479/1
  Constant_x_ddd_058ab/1 -> Subtract_9f2d1/1
  Constant_x_l_6bd17/1 -> Subtract_9f2d1/2
  Subtract_bd479/1 -> Divide_a7949/2
  State_psi_fd_SG_D_1_4a659/1 -> Product_aa5e2/1
  Constant_x_ddd_209e2/1 -> Divide_1490a/2
  Subtract_9f2d1/1 -> Product_aa5e2/2
  Product_74c8c/1 -> Subtract_e8463/2
  Constant_x_dd_3614c/1 -> Subtract_834dc/1
  Constant_x_l_35342/1 -> Subtract_834dc/2
  Subtract_834dc/1 -> Divide_39bf3/2
  Divide_39bf3/1 -> Subtract_aaa06/2
  Constant_R_a_a2592/1 -> Product_dfdca/1
  Subtract_aaa06/1 -> Product_dfdca/2
  MathFunc_cos_ec301/1 -> Product_0a1c5/2
  State_theta_SG_D_1_684aa/1 -> MathFunc_sin_a89c5/1
  Divide_1490a/1 -> Subtract_e8463/1
  Product_dfdca/1 -> Divide_1490a/1
  MathFunc_sin_a89c5/1 -> Product_74c8c/2
  Input_v_d_SG_D_1_7e265/1 -> Product_74c8c/1
  Product_b0c62/1 -> Blockout_d_psi_d_SG_D_1_08662/1
  Product_8bf94/1 -> Product_b0c62/1
  Product_e62b2/1 -> Product_8bf94/1
  State_theta_SG_D_1_1ab10/1 -> MathFunc_cos_ec301/1
  Constant_2.0_7bc02/1 -> Product_073ea/1
  Constant_pi_e16f2/1 -> Product_073ea/2
  Input_v_q_SG_D_1_b5510/1 -> Product_0a1c5/1
  Constant_f0_18599/1 -> Product_8bf94/2
  State_psi_q_SG_D_1_546c2/1 -> Product_b9ea6/1
  State_w_SG_D_1_cd758/1 -> Product_b9ea6/2
  Product_073ea/1 -> Product_a81f3/1
  Constant_pi_56cff/1 -> Product_e62b2/2
  Constant_f0_5b7b8/1 -> Product_a81f3/2
  Constant_-2.0_2801a/1 -> Product_e62b2/1
  Add_625df/1 -> Subtract_6b787/1
  Subtract_e8463/1 -> Add_625df/1
  Product_0a1c5/1 -> Add_625df/2
  Product_b9ea6/1 -> Divide_04fac/1
  Product_a81f3/1 -> Divide_04fac/2
  Divide_04fac/1 -> Subtract_6b787/2
  Subtract_6b787/1 -> Product_b0c62/2

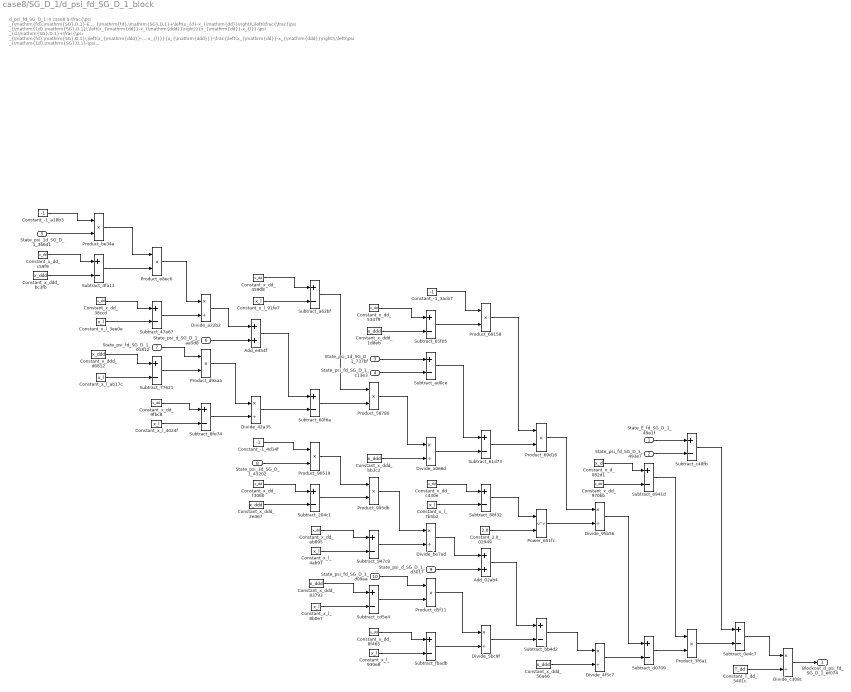
== system case8/SG_D_1/d_psi_fd_SG_D_1_block ==
  note: d_psi_fd_SG_D_1 in case8
      | $-\frac{\psi _{\mathrm{fd},\mathrm{SG},D,1}-E_{\mathrm{fd},\mathrm{SG},D,1}+\left(x_{d}-x_{\mathrm{dd}}\right)\,\left(\frac{\frac{\psi _{\mathrm{1d},\mathrm{SG},D,1}\,\left(x_{\mathrm{dd}}-x_{\mathrm{ddd}}\right)}{x_{\mathrm{dd}}-x_{l}}-\psi _{d,\mathrm{SG},D,1}+\frac{\psi _{\mathrm{fd},\mathrm{SG},D,1}\,\left(x_{\mathrm{ddd}}-x_{l}\right)}{x_{\mathrm{dd}}-x_{l}}}{x_{\mathrm{ddd}}}-\frac{\left(x_{\mathrm{dd}}-x_{\mathrm{ddd}}\right)\,\left(\psi _{\mathrm{1d},\mathrm{SG},D,1}-\psi _{\mathrm{fd},\mathrm{SG},D,1}+\frac{\left(x_{\mathrm{dd}}-x_{l}\right)\,\left(\frac{\psi _{\mathrm{1d},\mathrm{SG},D,1}\,\left(x_{\mathrm{dd}}-x_{\mathrm{ddd}}\right)}{x_{\mathrm{dd}}-x_{l}}-\psi _{d,\mathrm{SG},D,1}+\frac{\psi _{\mathrm{fd},\mathrm{SG},D,1}\,\left(x_{\mathrm{ddd}}-x_{l}\right)}{x_{\mathrm{dd}}-x_{l}}\right)}{x_{\mathrm{ddd}}}\right)}{{\left(x_{\mathrm{dd}}-x_{l}\right)}^2}\right)}{T_{\mathrm{dd}}}$
      | Automatically generated on 2025-10-31 19:29:32 .
  State_E_fd_SG_D_1_49e1f : Inport
  State_psi_fd_SG_D_1_493e7 : Inport  Port=2
  State_psi_1d_SG_D_1_737bf : Inport  Port=3
  State_psi_fd_SG_D_1_c13e3 : Inport  Port=4
  State_psi_1d_SG_D_1_36641 : Inport  Port=5
  State_psi_d_SG_D_1_aa5d8 : Inport  Port=6
  State_psi_fd_SG_D_1_01812 : Inport  Port=7
  State_psi_1d_SG_D_1_43202 : Inport  Port=8
  State_psi_d_SG_D_1_d3017 : Inport  Port=9
  State_psi_fd_SG_D_1_d09aa : Inport  Port=10
  Add_02ab4 : Sum
  Add_e454f : Sum
  Constant_-1_3acb7 : Constant  Value=-1
  Constant_-1_4d14f : Constant  Value=-1
  Constant_-1_a18b3 : Constant  Value=-1
  Constant_2.0_02949 : Constant  Value=2.0
  Constant_T_dd_5401c : Constant  Value=T_dd
  Constant_x_d_082d1 : Constant  Value=x_d
  Constant_x_dd_38ccd : Constant  Value=x_dd
  Constant_x_dd_45908 : Constant  Value=x_dd
  Constant_x_dd_53479 : Constant  Value=x_dd
  Constant_x_dd_8f465 : Constant  Value=x_dd
  Constant_x_dd_970bb : Constant  Value=x_dd
  Constant_x_dd_9fbc8 : Constant  Value=x_dd
  Constant_x_dd_ab895 : Constant  Value=x_dd
  Constant_x_dd_c430e : Constant  Value=x_dd
  Constant_x_dd_c59f9 : Constant  Value=x_dd
  Constant_x_dd_f3060 : Constant  Value=x_dd
  Constant_x_ddd_1d8eb : Constant  Value=x_ddd
  Constant_x_ddd_2e467 : Constant  Value=x_ddd
  Constant_x_ddd_56a66 : Constant  Value=x_ddd
  Constant_x_ddd_83793 : Constant  Value=x_ddd
  Constant_x_ddd_bb3c2 : Constant  Value=x_ddd
  Constant_x_ddd_bc3fb : Constant  Value=x_ddd
  Constant_x_ddd_d6812 : Constant  Value=x_ddd
  Constant_x_l_3ee0e : Constant  Value=x_l
  Constant_x_l_4024f : Constant  Value=x_l
  Constant_x_l_4ab97 : Constant  Value=x_l
  Constant_x_l_7b5b2 : Constant  Value=x_l
  Constant_x_l_8b0e7 : Constant  Value=x_l
  Constant_x_l_91fe7 : Constant  Value=x_l
  Constant_x_l_930e8 : Constant  Value=x_l
  Constant_x_l_ab17c : Constant  Value=x_l
  Divide_42a35 : Product  Inputs=*/
  Divide_4f5c7 : Product  Inputs=*/
  Divide_5bc9f : Product  Inputs=*/
  Divide_95b56 : Product  Inputs=*/
  Divide_a066d : Product  Inputs=*/
  Divide_a22b2 : Product  Inputs=*/
  Divide_be7ad : Product  Inputs=*/
  Divide_c308c : Product  Inputs=*/
  Power_651fc : Math  Operator=pow
  Product_3f6a1 : Product
  Product_58780 : Product
  Product_69158 : Product
  Product_69d16 : Product
  Product_90519 : Product
  Product_995db : Product
  Product_be34a : Product
  Product_d5f11 : Product
  Product_d9aaa : Product
  Product_e8ec6 : Product
  Subtract_0e4c7 : Sum  Inputs=+-
  Subtract_204c1 : Sum  Inputs=+-
  Subtract_47a67 : Sum  Inputs=+-
  Subtract_4fa11 : Sum  Inputs=+-
  Subtract_60f6a : Sum  Inputs=+-
  Subtract_61d73 : Sum  Inputs=+-
  Subtract_65f05 : Sum  Inputs=+-
  Subtract_77621 : Sum  Inputs=+-
  Subtract_88f32 : Sum  Inputs=+-
  Subtract_8fe74 : Sum  Inputs=+-
  Subtract_947c8 : Sum  Inputs=+-
  Subtract_a62bf : Sum  Inputs=+-
  Subtract_ad0ce : Sum  Inputs=+-
  Subtract_bb4d2 : Sum  Inputs=+-
  Subtract_c48fb : Sum  Inputs=+-
  Subtract_cd5e4 : Sum  Inputs=+-
  Subtract_d0709 : Sum  Inputs=+-
  Subtract_e941d : Sum  Inputs=+-
  Subtract_fbadb : Sum  Inputs=+-
  Blockout_d_psi_fd_SG_D_1_ef074 : Outport
  wires:
  State_psi_d_SG_D_1_aa5d8/1 -> Add_e454f/2
  Constant_x_dd_38ccd/1 -> Subtract_47a67/1
  Product_e8ec6/1 -> Divide_a22b2/1
  Subtract_4fa11/1 -> Product_e8ec6/2
  Subtract_60f6a/1 -> Product_58780/2
  Product_be34a/1 -> Product_e8ec6/1
  Constant_x_dd_c59f9/1 -> Subtract_4fa11/1
  Constant_x_l_91fe7/1 -> Subtract_a62bf/2
  Constant_-1_a18b3/1 -> Product_be34a/1
  Subtract_a62bf/1 -> Product_58780/1
  Constant_x_l_3ee0e/1 -> Subtract_47a67/2
  Constant_x_ddd_bc3fb/1 -> Subtract_4fa11/2
  State_psi_1d_SG_D_1_36641/1 -> Product_be34a/2
  Constant_x_ddd_d6812/1 -> Subtract_77621/1
  Constant_x_l_ab17c/1 -> Subtract_77621/2
  State_E_fd_SG_D_1_49e1f/1 -> Subtract_c48fb/1
  Divide_a22b2/1 -> Add_e454f/1
  Subtract_47a67/1 -> Divide_a22b2/2
  State_psi_fd_SG_D_1_01812/1 -> Product_d9aaa/1
  Constant_x_ddd_bb3c2/1 -> Divide_a066d/2
  Subtract_77621/1 -> Product_d9aaa/2
  Constant_x_dd_9fbc8/1 -> Subtract_8fe74/1
  Constant_x_dd_c430e/1 -> Subtract_88f32/1
  State_psi_fd_SG_D_1_493e7/1 -> Subtract_c48fb/2
  Constant_x_l_4024f/1 -> Subtract_8fe74/2
  Product_d9aaa/1 -> Divide_42a35/1
  Constant_-1_3acb7/1 -> Product_69158/1
  Subtract_8fe74/1 -> Divide_42a35/2
  Constant_x_dd_45908/1 -> Subtract_a62bf/1
  Add_e454f/1 -> Subtract_60f6a/1
  Constant_x_l_7b5b2/1 -> Subtract_88f32/2
  Divide_42a35/1 -> Subtract_60f6a/2
  Divide_95b56/1 -> Subtract_d0709/1
  Constant_-1_4d14f/1 -> Product_90519/1
  State_psi_1d_SG_D_1_43202/1 -> Product_90519/2
  Constant_x_dd_f3060/1 -> Subtract_204c1/1
  Subtract_65f05/1 -> Product_69158/2
  Constant_x_ddd_2e467/1 -> Subtract_204c1/2
  Product_90519/1 -> Product_995db/1
  Constant_2.0_02949/1 -> Power_651fc/2
  Product_995db/1 -> Divide_be7ad/1
  Subtract_d0709/1 -> Product_3f6a1/2
  Subtract_204c1/1 -> Product_995db/2
  State_psi_d_SG_D_1_d3017/1 -> Add_02ab4/2
  Constant_x_dd_ab895/1 -> Subtract_947c8/1
  Constant_x_l_4ab97/1 -> Subtract_947c8/2
  Constant_x_dd_53479/1 -> Subtract_65f05/1
  Divide_a066d/1 -> Subtract_61d73/2
  Constant_x_ddd_83793/1 -> Subtract_cd5e4/1
  Constant_x_ddd_1d8eb/1 -> Subtract_65f05/2
  Constant_x_l_8b0e7/1 -> Subtract_cd5e4/2
  Subtract_cd5e4/1 -> Product_d5f11/2
  State_psi_1d_SG_D_1_737bf/1 -> Subtract_ad0ce/1
  Product_d5f11/1 -> Divide_5bc9f/1
  State_psi_fd_SG_D_1_c13e3/1 -> Subtract_ad0ce/2
  State_psi_fd_SG_D_1_d09aa/1 -> Product_d5f11/1
  Product_58780/1 -> Divide_a066d/1
  Divide_be7ad/1 -> Add_02ab4/1
  Subtract_947c8/1 -> Divide_be7ad/2
  Constant_x_dd_8f465/1 -> Subtract_fbadb/1
  Constant_x_l_930e8/1 -> Subtract_fbadb/2
  Divide_5bc9f/1 -> Subtract_bb4d2/2
  Subtract_ad0ce/1 -> Subtract_61d73/1
  Subtract_fbadb/1 -> Divide_5bc9f/2
  Subtract_61d73/1 -> Product_69d16/2
  Product_69158/1 -> Product_69d16/1
  Subtract_88f32/1 -> Power_651fc/1
  Add_02ab4/1 -> Subtract_bb4d2/1
  Product_69d16/1 -> Divide_95b56/1
  Power_651fc/1 -> Divide_95b56/2
  Subtract_bb4d2/1 -> Divide_4f5c7/1
  Constant_x_ddd_56a66/1 -> Divide_4f5c7/2
  Constant_x_d_082d1/1 -> Subtract_e941d/1
  Constant_x_dd_970bb/1 -> Subtract_e941d/2
  Divide_4f5c7/1 -> Subtract_d0709/2
  Subtract_e941d/1 -> Product_3f6a1/1
  Subtract_c48fb/1 -> Subtract_0e4c7/1
  Product_3f6a1/1 -> Subtract_0e4c7/2
  Subtract_0e4c7/1 -> Divide_c308c/1
  Constant_T_dd_5401c/1 -> Divide_c308c/2
  Divide_c308c/1 -> Blockout_d_psi_fd_SG_D_1_ef074/1

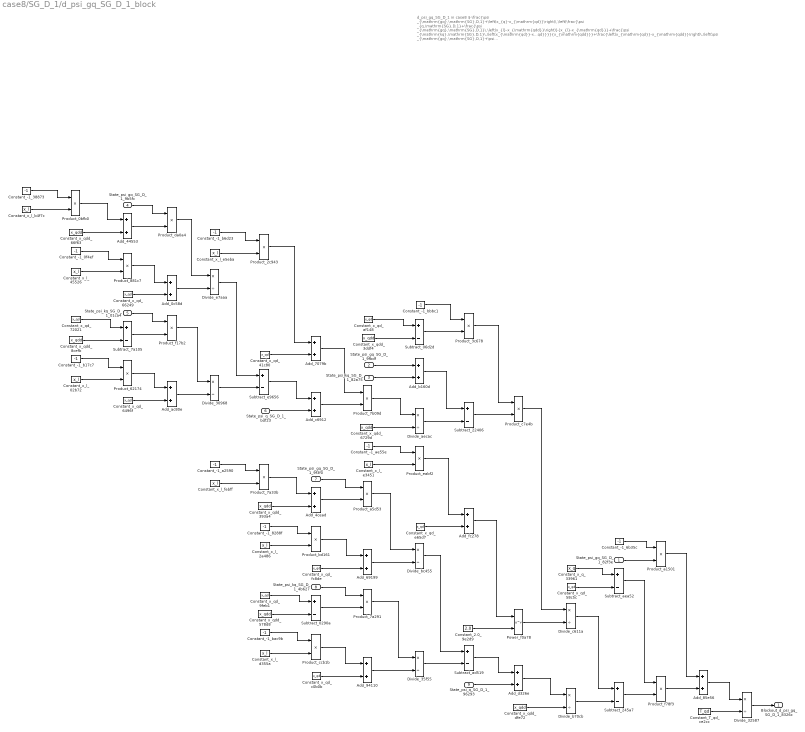
== system case8/SG_D_1/d_psi_gq_SG_D_1_block ==
  note: d_psi_gq_SG_D_1 in case8
      | $-\frac{\psi _{\mathrm{gq},\mathrm{SG},D,1}+\left(x_{q}-x_{\mathrm{qd}}\right)\,\left(\frac{\psi _{q,\mathrm{SG},D,1}+\frac{\psi _{\mathrm{gq},\mathrm{SG},D,1}\,\left(x_{l}-x_{\mathrm{qdd}}\right)}{x_{l}-x_{\mathrm{qd}}}+\frac{\psi _{\mathrm{kq},\mathrm{SG},D,1}\,\left(x_{\mathrm{qd}}-x_{\mathrm{qdd}}\right)}{x_{l}-x_{\mathrm{qd}}}}{x_{\mathrm{qdd}}}+\frac{\left(x_{\mathrm{qd}}-x_{\mathrm{qdd}}\right)\,\left(\psi _{\mathrm{gq},\mathrm{SG},D,1}+\psi _{\mathrm{kq},\mathrm{SG},D,1}+\frac{\left(x_{l}-x_{\mathrm{qd}}\right)\,\left(\psi _{q,\mathrm{SG},D,1}+\frac{\psi _{\mathrm{gq},\mathrm{SG},D,1}\,\left(x_{l}-x_{\mathrm{qdd}}\right)}{x_{l}-x_{\mathrm{qd}}}+\frac{\psi _{\mathrm{kq},\mathrm{SG},D,1}\,\left(x_{\mathrm{qd}}-x_{\mathrm{qdd}}\right)}{x_{l}-x_{\mathrm{qd}}}\right)}{x_{\mathrm{qdd}}}\right)}{{\left(x_{l}-x_{\mathrm{qd}}\right)}^2}\right)}{T_{\mathrm{qd}}}$
      | Automatically generated on 2025-10-31 19:29:34 .
  State_psi_gq_SG_D_1_82f3e : Inport
  State_psi_gq_SG_D_1_9fbdf : Inport  Port=2
  State_psi_kq_SG_D_1_82a75 : Inport  Port=3
  State_psi_gq_SG_D_1_9b5fc : Inport  Port=4
  State_psi_kq_SG_D_1_01ca4 : Inport  Port=5
  State_psi_q_SG_D_1_bdf23 : Inport  Port=6
  State_psi_gq_SG_D_1_9f3f0 : Inport  Port=7
  State_psi_kq_SG_D_1_4b627 : Inport  Port=8
  State_psi_q_SG_D_1_96293 : Inport  Port=9
  Add_0c58d : Sum
  Add_44553 : Sum
  Add_4cead : Sum
  Add_69199 : Sum
  Add_7079b : Sum
  Add_85e56 : Sum
  Add_94110 : Sum
  Add_ac80e : Sum
  Add_b160d : Sum
  Add_c6912 : Sum
  Add_d326e : Sum
  Add_fc278 : Sum
  Constant_-1_0f4ef : Constant  Value=-1
  Constant_-1_38873 : Constant  Value=-1
  Constant_-1_6b35c : Constant  Value=-1
  Constant_-1_8288f : Constant  Value=-1
  Constant_-1_a2590 : Constant  Value=-1
  Constant_-1_ae55e : Constant  Value=-1
  Constant_-1_b17c7 : Constant  Value=-1
  Constant_-1_b6d23 : Constant  Value=-1
  Constant_-1_bac9b : Constant  Value=-1
  Constant_-1_bbbc1 : Constant  Value=-1
  Constant_2.0_9e2d9 : Constant  Value=2.0
  Constant_T_qd_ce2cc : Constant  Value=T_qd
  Constant_x_l_02b72 : Constant  Value=x_l
  Constant_x_l_2a486 : Constant  Value=x_l
  Constant_x_l_45526 : Constant  Value=x_l
  Constant_x_l_b4f7c : Constant  Value=x_l
  Constant_x_l_d355a : Constant  Value=x_l
  Constant_x_l_e3451 : Constant  Value=x_l
  Constant_x_l_e5eba : Constant  Value=x_l
  Constant_x_l_febff : Constant  Value=x_l
  Constant_x_q_33961 : Constant  Value=x_q
  Constant_x_qd_41c80 : Constant  Value=x_qd
  Constant_x_qd_58c5c : Constant  Value=x_qd
  Constant_x_qd_6496f : Constant  Value=x_qd
  Constant_x_qd_66249 : Constant  Value=x_qd
  Constant_x_qd_72021 : Constant  Value=x_qd
  Constant_x_qd_9feb1 : Constant  Value=x_qd
  Constant_x_qd_af148 : Constant  Value=x_qd
  Constant_x_qd_c0b0b : Constant  Value=x_qd
  Constant_x_qd_e65d7 : Constant  Value=x_qd
  Constant_x_qd_fc8de : Constant  Value=x_qd
  Constant_x_qdd_393a4 : Constant  Value=x_qdd
  Constant_x_qdd_3ddf4 : Constant  Value=x_qdd
  Constant_x_qdd_578d8 : Constant  Value=x_qdd
  Constant_x_qdd_66f63 : Constant  Value=x_qdd
  Constant_x_qdd_6729d : Constant  Value=x_qdd
  Constant_x_qdd_8cefb : Constant  Value=x_qdd
  Constant_x_qdd_dfe72 : Constant  Value=x_qdd
  Divide_30968 : Product  Inputs=*/
  Divide_32587 : Product  Inputs=*/
  Divide_35f55 : Product  Inputs=*/
  Divide_aecac : Product  Inputs=*/
  Divide_b70cb : Product  Inputs=*/
  Divide_bc455 : Product  Inputs=*/
  Divide_c611a : Product  Inputs=*/
  Divide_e7aaa : Product  Inputs=*/
  Power_f0a78 : Math  Operator=pow
  Product_0bfb0 : Product
  Product_2c943 : Product
  Product_3c678 : Product
  Product_62174 : Product
  Product_7a291 : Product
  Product_7a33b : Product
  Product_7b09d : Product
  Product_881c7 : Product
  Product_a1501 : Product
  Product_a5d53 : Product
  Product_bd161 : Product
  Product_c7e4b : Product
  Product_ccb1b : Product
  Product_da0a4 : Product
  Product_eabf2 : Product
  Product_f17b2 : Product
  Product_f78f3 : Product
  Subtract_0290a : Sum  Inputs=+-
  Subtract_06d2d : Sum  Inputs=+-
  Subtract_22406 : Sum  Inputs=+-
  Subtract_245a7 : Sum  Inputs=+-
  Subtract_7a105 : Sum  Inputs=+-
  Subtract_ad519 : Sum  Inputs=+-
  Subtract_aea52 : Sum  Inputs=+-
  Subtract_e9656 : Sum  Inputs=+-
  Blockout_d_psi_gq_SG_D_1_8326c : Outport
  wires:
  State_psi_gq_SG_D_1_9b5fc/1 -> Product_da0a4/1
  Constant_-1_0f4ef/1 -> Product_881c7/1
  Divide_e7aaa/1 -> Subtract_e9656/1
  Add_0c58d/1 -> Divide_e7aaa/2
  Product_0bfb0/1 -> Add_44553/1
  Constant_x_qd_41c80/1 -> Add_7079b/2
  Constant_-1_38873/1 -> Product_0bfb0/1
  Constant_x_qdd_66f63/1 -> Add_44553/2
  Constant_x_l_45526/1 -> Product_881c7/2
  Constant_x_l_b4f7c/1 -> Product_0bfb0/2
  Constant_-1_b17c7/1 -> Product_62174/1
  Constant_x_qd_72021/1 -> Subtract_7a105/1
  Constant_x_qdd_6729d/1 -> Divide_aecac/2
  Constant_x_l_02b72/1 -> Product_62174/2
  Constant_x_qdd_8cefb/1 -> Subtract_7a105/2
  Subtract_e9656/1 -> Add_c6912/1
  Add_44553/1 -> Product_da0a4/2
  Product_da0a4/1 -> Divide_e7aaa/1
  Product_881c7/1 -> Add_0c58d/1
  Constant_x_qd_66249/1 -> Add_0c58d/2
  State_psi_kq_SG_D_1_01ca4/1 -> Product_f17b2/1
  Product_62174/1 -> Add_ac80e/1
  Subtract_7a105/1 -> Product_f17b2/2
  Constant_x_qd_6496f/1 -> Add_ac80e/2
  Product_f17b2/1 -> Divide_30968/1
  Add_ac80e/1 -> Divide_30968/2
  Constant_-1_bbbc1/1 -> Product_3c678/1
  Constant_-1_b6d23/1 -> Product_2c943/1
  Add_69199/1 -> Divide_bc455/2
  Product_ccb1b/1 -> Add_94110/1
  Subtract_0290a/1 -> Product_7a291/2
  Constant_x_l_e5eba/1 -> Product_2c943/2
  Divide_30968/1 -> Subtract_e9656/2
  Subtract_aea52/1 -> Product_f78f3/1
  Constant_-1_ae55e/1 -> Product_eabf2/1
  Constant_-1_a2590/1 -> Product_7a33b/1
  Constant_x_l_e3451/1 -> Product_eabf2/2
  Constant_x_l_febff/1 -> Product_7a33b/2
  Constant_x_qd_fc8de/1 -> Add_69199/2
  Product_2c943/1 -> Add_7079b/1
  State_psi_q_SG_D_1_bdf23/1 -> Add_c6912/2
  Product_7a33b/1 -> Add_4cead/1
  Constant_x_qdd_393a4/1 -> Add_4cead/2
  Constant_-1_8288f/1 -> Product_bd161/1
  Constant_x_qd_c0b0b/1 -> Add_94110/2
  Add_7079b/1 -> Product_7b09d/1
  Constant_x_l_2a486/1 -> Product_bd161/2
  Constant_-1_bac9b/1 -> Product_ccb1b/1
  Constant_x_qd_9feb1/1 -> Subtract_0290a/1
  Product_7b09d/1 -> Divide_aecac/1
  Constant_x_l_d355a/1 -> Product_ccb1b/2
  Divide_c611a/1 -> Subtract_245a7/1
  Constant_x_qdd_578d8/1 -> Subtract_0290a/2
  Add_c6912/1 -> Product_7b09d/2
  State_psi_gq_SG_D_1_9f3f0/1 -> Product_a5d53/1
  Add_4cead/1 -> Product_a5d53/2
  Product_bd161/1 -> Add_69199/1
  State_psi_kq_SG_D_1_4b627/1 -> Product_7a291/1
  Add_94110/1 -> Divide_35f55/2
  State_psi_gq_SG_D_1_9fbdf/1 -> Add_b160d/1
  Constant_x_qd_af148/1 -> Subtract_06d2d/1
  Constant_x_qdd_3ddf4/1 -> Subtract_06d2d/2
  Product_7a291/1 -> Divide_35f55/1
  State_psi_kq_SG_D_1_82a75/1 -> Add_b160d/2
  Product_a5d53/1 -> Divide_bc455/1
  Subtract_06d2d/1 -> Product_3c678/2
  Add_b160d/1 -> Subtract_22406/1
  Divide_aecac/1 -> Subtract_22406/2
  Product_eabf2/1 -> Add_fc278/1
  Constant_x_qd_e65d7/1 -> Add_fc278/2
  Divide_bc455/1 -> Subtract_ad519/1
  Divide_35f55/1 -> Subtract_ad519/2
  Product_3c678/1 -> Product_c7e4b/1
  Subtract_22406/1 -> Product_c7e4b/2
  Add_fc278/1 -> Power_f0a78/1
  Constant_2.0_9e2d9/1 -> Power_f0a78/2
  Subtract_ad519/1 -> Add_d326e/1
  State_psi_q_SG_D_1_96293/1 -> Add_d326e/2
  Product_c7e4b/1 -> Divide_c611a/1
  Power_f0a78/1 -> Divide_c611a/2
  Add_d326e/1 -> Divide_b70cb/1
  Constant_x_qdd_dfe72/1 -> Divide_b70cb/2
  Constant_x_q_33961/1 -> Subtract_aea52/1
  Constant_x_qd_58c5c/1 -> Subtract_aea52/2
  Divide_b70cb/1 -> Subtract_245a7/2
  Constant_-1_6b35c/1 -> Product_a1501/1
  State_psi_gq_SG_D_1_82f3e/1 -> Product_a1501/2
  Subtract_245a7/1 -> Product_f78f3/2
  Product_a1501/1 -> Add_85e56/1
  Product_f78f3/1 -> Add_85e56/2
  Add_85e56/1 -> Divide_32587/1
  Constant_T_qd_ce2cc/1 -> Divide_32587/2
  Divide_32587/1 -> Blockout_d_psi_gq_SG_D_1_8326c/1
